simulink model "Elektrodeionisatior_R2024b"  (R2024b)
settings: Solver=VariableStepAuto  StartTime=0.0  StopTime=10.0  RelTol=1e-3
settings Model: Creator=Jan.Seemann  LastModifiedBy=Jan.Seemann

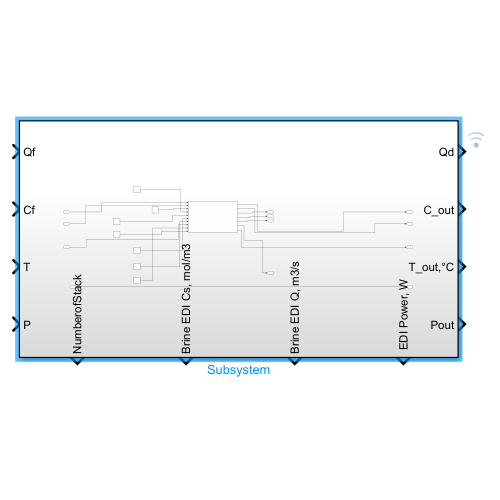
[thumbnail: Simulink's stored preview of the top-level diagram]
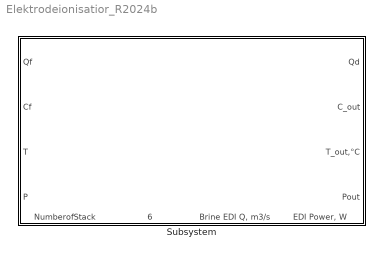
== system Elektrodeionisatior_R2024b ==
  Subsystem : Subsystem
      settings: PortSchema="{\"entries\":[{\"content\":{\"sides\":[{\"content\":{\"connectorIds\":[\"In1\",\"In2\",\"In3\",\"In4\"]},\"type\":\"ConnectorPlacement.EquallySpacedRectSide\",\"uuid\":\"8127a076-605d-4ed1-91b0-972f77442893\"},{\"content\":{\"connectorIds\":[\"Out1\",\"Out2\",\"Out3\",\"Out4\"],\"side\":\"RIGHT\"},\"type\":\"ConnectorPlacement.EquallySpacedRectSide\",\"uuid\":\"a8fe5e60-1d23-4e07-8145-0361b63bfa06\"},{\"content\":{\"side\":\"TOP\"},\"type\":\"ConnectorPlacement.EquallySpacedRectSide\",\"uuid\":\"b42cffd3-1fd8-4869-a126-4ae6a788e324\"},{\"content\":{\"connectorIds\":[\"Out5\",\"Out6\",\"Out7\",\"Out8\"],\"side\":\"BOTTOM\"},\"type\":\"ConnectorPlacement.EquallySpacedRectSide\",\"uuid\":\"bd13aaa3-40d7-41f8-8bf0-7622a41931bd\"}]},\"type\":\"ConnectorPlacement.EquallySpacedConnector\",\"uuid\":\"080b4185-89f1-45ca-abee-f0e4dfd2aadb\"}],\"packageUris\":[\"http://schema.mathworks.com/mf0/Connector/R2020b\"],\"version\":\"1.0\"}"

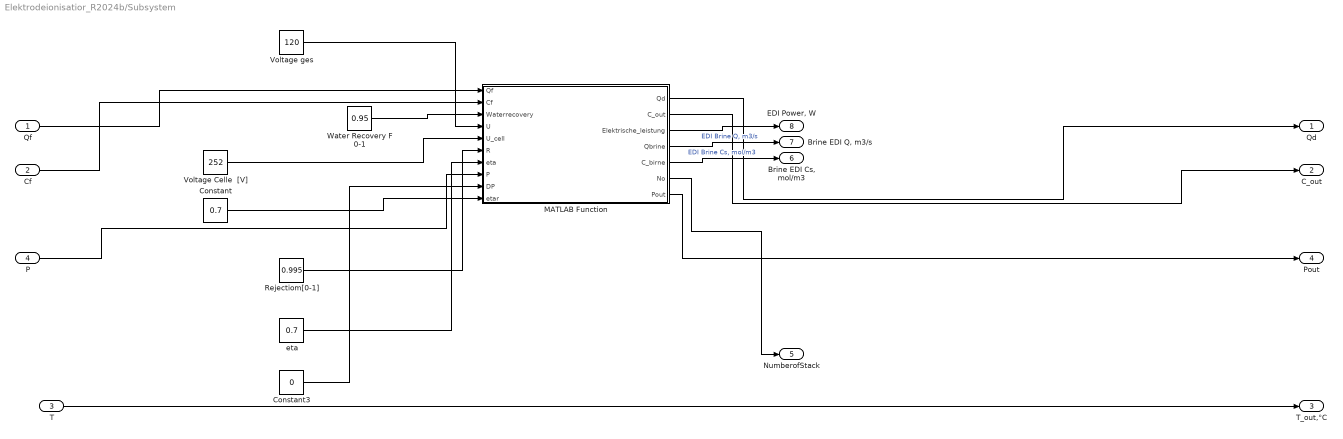
== system Elektrodeionisatior_R2024b/Subsystem ==
  Qf : Inport
  Cf : Inport  Port=2
  T : Inport  Port=3
  P : Inport  Port=4
  Constant : Constant  Value=0.7
  Constant3 : Constant  Value=0
  MATLAB Function : MATLAB Function  TreatAsAtomicUnit=on
  Rejectiom[0-1] : Constant  Value=0.995
  Voltage Celle  [V] : Constant  Value=252
  Voltage ges : Constant  Value=120
  Water Recovery F 0-1 : Constant  Value=0.95
  "eta " : Constant  Value=0.7
  Qd : Outport
  C_out : Outport  Port=2
  T_out,°C : Outport  Port=3
  Pout : Outport  Port=4
  NumberofStack : Outport  Port=5
  "Brine EDI Cs, mol/m3" : Outport  Port=6
  "Brine EDI Q, m3/s " : Outport  Port=7
  " EDI Power, W" : Outport  Port=8
  wires:
  MATLAB Function/6(No) -> NumberofStack/1
  Water Recovery F 0-1/1 -> MATLAB Function/3(Waterrecovery)
  MATLAB Function/5(C_birne) -> "Brine EDI Cs, mol/m3"/1  "EDI Brine Cs, mol/m3"
  MATLAB Function/7(Pout) -> Pout/1
  Voltage ges/1 -> MATLAB Function/4(U)
  Cf/1 -> MATLAB Function/2(Cf)
  Rejectiom[0-1]/1 -> MATLAB Function/6(R)
  P/1 -> MATLAB Function/8(P)
  Constant3/1 -> MATLAB Function/9(DP)
  Voltage Celle  [V]/1 -> MATLAB Function/5(U_cell)
  "eta "/1 -> MATLAB Function/7(eta)
  MATLAB Function/1(Qd) -> Qd/1
  MATLAB Function/3(Elektrische_leistung) -> " EDI Power, W"/1
  MATLAB Function/4(Qbrine) -> "Brine EDI Q, m3/s "/1  "EDI Brine Q, m3/s"
  Qf/1 -> MATLAB Function/1(Qf)
  MATLAB Function/2(C_out) -> C_out/1
  Constant/1 -> MATLAB Function/10(etar)
  T/1 -> T_out,°C/1

== matlab function Elektrodeionisatior_R2024b/Subsystem/MATLAB Function ==
  data: Qf input; Cf input; Waterrecovery input; U input; U_cell input; R input; eta input; Qd output; C_out output; Elektrische_leistung output; Qbrine output; C_birne output; No output; P input; DP input; Pout output; etar input
function [Qd, C_out,Elektrische_leistung,Qbrine,C_birne, No, Pout] = EDI_cal ( Qf,Cf,Waterrecovery, U, U_cell,R, eta, P , DP, etar)
    
    % Autor Jan Seemann 21.11.2024 
    %% Quellen 
    % Emprisches Model basierenden auf den Daten von Liu et al (2007) doi:10.1016/j.desal.2007.01.102
    % die Eingabe Parameter sind wie Folgt definiert 
    % Continuous Electrodeionization - von Jonathan H. Wood and Joseph D. Gifford 
    % Jane Kucera (ed.) Desalination 2nd Edition, (287–328) © 2019 Scrivener Publishing LLC
    % 
    %% _______ Inputs_______
    %Rejection von Salz
    % R = 0.99; 
    % %Waterrecoveryrate 
    % Waterrecovery = 0.9;
    % %Stromwirkungsgrad, als Bruch (dimensionslos)
    % eta = 0.97;
    % % Inlet flow in m3/h 
    % Qf = 0.4;
    % % Salzgehalt in mg/L
    % Cf = 1.23;
    % % Spannung pro Zelle
    % U_cell = 5; % V 
    % % Gesammtspannung
    % U = 400; %V
    % % Anzahl Stack
    

    %% Physikalische Eigenschaften
    % Molaremasse von NaCl
    MNacl = 58.44 ;%g/mol
    % Faraday-Konstante
    F = 96487 ; % As
    
    
    %% Berechnung 
    %% Wasserstrom berechnnung
    Qd = Qf * Waterrecovery;
    %% Bestimmun der Differenz von Inlet Konzentration und Outlet KOnzentrartion
    Cdi = R * Cf; % mg/L
    % C_out bestimmen
    C_out = Cf -  Cdi ;
    % Umwandel der einheit der Startkonzentration in mol/L
    Cdi = Cdi / 1000 / MNacl;
    % Brine 
    Qbrine = Qf-Qd;
    C_birne = Cf-C_out;
    %% Bestimmung der tatsächlicher Gleichstrom, der einem CEDI-Modul zugeführt wird, in Ampere
    No = U/ U_cell ; % Number of Stack
    % Bestimmung der Stromstärke
    Ia = F * (Cdi) * Qd/ ( eta * No * 3600 )*1000 ; % As/mol * mol/L * m3/h *h/3600s *1000L/m3 = A  
    % Bestimmung der Elektrischen_Leistung 
    Elektrische_leistung = Ia * U_cell * No /etar ;% V * I = W
    
    % Bestimmung der Elektrischen-Leitung per Voulumenstrom
    Elektrische_leistung_per_flow = Elektrische_leistung / Qf *1000; % kWh/m3
    %% Druckverlust
    Pout = P- DP;



end
